simulink model "Estancia2024_2022a"  (R2022a)
settings: Solver=ode1  StartTime=0.0  StopTime=inf  FixedStep=0.0025  RelTol=1e-3  EnableMultiTasking=on
InitFcn:
  | Motor_Mapping_7_Inch
model workspace (MAT data in the model file):
  target_system = 1
values from neighbouring files (symbols this model uses):
  F1 = F1 + 2*(PSI_I'*C'*Q_z*C*PHI_I)    [Setup_MPC_SMC_Drone.m]
  F1_xy = F1_xy + 2*(PSI_xy_I'*C_xy'*Q_xy*C_xy*PHI_xy_I)    [Setup_MPC_SMC_Drone.m]
  F2 = F2 - 2*(PSI_I'*C'*Q_z*pi_n)    [Setup_MPC_SMC_Drone.m]
  F2_xy = F2_xy - 2*(PSI_xy_I'*C_xy'*Q_xy*pi_n)    [Setup_MPC_SMC_Drone.m]
  F3 = F3 - 2*(pi_nu'*Qt_z)    [Setup_MPC_SMC_Drone.m]
  F3_xy = F3_xy - 2*(pi_nu'*R_xy)    [Setup_MPC_SMC_Drone.m]
  F4 = F4 + 2*(PSI_I'*C'*Qt_z*C*SumG)    [Setup_MPC_SMC_Drone.m]
  G = [0;-g]    [Setup_MPC_SMC_Drone.m]
  H = H + 2*(PSI_I'*C'*Q_z*C*PSI_I + pi_nu'*Qt_z*pi_nu)    [Setup_MPC_SMC_Drone.m]
  H_xy = H_xy + 2*(PSI_xy_I'*C_xy'*Q_xy*C_xy*PSI_xy_I + pi_nu'*R_xy*pi_nu)    [Setup_MPC_SMC_Drone.m]
  J = diag([Jxx Jyy Jzz])    [Setup_MPC_SMC_Drone.m]
  m = 1.121    [Setup_MPC_SMC_Drone.m]
  N = 10    [Setup_MPC_SMC_Drone.m]
  N_xy = 10    [Setup_MPC_SMC_Drone.m]
  ny = size(C,1)    [Setup_MPC_SMC_Drone.m]
  ny_xy = size(C_xy,1)    [Setup_MPC_SMC_Drone.m]
  u_des = 0    [Setup_MPC_SMC_Drone.m]
  u_des_xy = [0;0]    [Setup_MPC_SMC_Drone.m]
undefined symbols (not defined in the file or in its folder): _Commander, _QDrone2, _Stabilizer, A_l, B_l, C_l, datetime, F1_l, F1_z, F2_l, F2_z, F3_l, F3_z, F4_z, H_l, H_z, HIL, KT, lf, log_, max_ul, min_ul, Motor_Matrix, n, N_l, N_z, nr_l, nr_z, nu, nu_l, nu_xy, nu_z, phi_l, psi_l, qc_get_step_size, Qu_l, Qy_l, s, saved_data, u_dz, ud_l
libraries: quarc_library x95, simulink x27, simulink_extras x10, matrix_library x1, aerolibutil x1
(part 4 of 5)

== system Estancia2024_2022a/COMMANDER (ANGLE MODE)/Subsystem/Z MPC ==
  pose : Inport
  pose_rate : Inport  Port=2
  ref : Inport  Port=3
  Add : Sum  Inputs=+++-
  Add1 : Sum
  Constant : Constant  Value=F1
  Constant1 : Constant  Value=F2
  Constant2 : Constant  Value=F3
  Constant3 : Constant  Value=F4
  Constant4 : Constant  Value=H
  Constant5 : Constant  Value=u_des
  Constant6 : Constant  Commented=on  Value=G
  Constant7 : Constant  Value=ones(1,N)
  Constant8 : Constant  Commented=on  Value=ones(2,N*2)
  Constant9 : Constant  Value=0.38
  MATLAB Function : MATLAB Function  TreatAsAtomicUnit=on
  MATLAB Function1 : MATLAB Function  Commented=on  TreatAsAtomicUnit=on
  MatrixMultiply{,1..3} (4 alike) : Product  Multiplication=Matrix(*)
  MatrixMultiply5 : Product  Commented=on  Multiplication=Matrix(*)
  Mux : Mux  Inputs=2
  Product : Product
  Reshape : Reshape  OutputDimensionality=Customize  OutputDimensions=[N*ny,1]
  Reshape1 : Reshape  Commented=on  OutputDimensionality=Customize  OutputDimensions=[2*N,1]
  Saturation : Saturate  UpperLimit=50  LowerLimit=0
  Scope : Scope
  Selector : Selector  InputPortWidth=N*nu  IndexOptions=Index vector (dialog)  Indices=1  OutputSizes=1
  Selector1 : Selector  InputPortWidth=4  IndexOptions=Index vector (dialog)  Indices=3  OutputSizes=1
  Selector2 : Selector  InputPortWidth=4  IndexOptions=Index vector (dialog)  Indices=3  OutputSizes=1
  Selector3 : Selector  InputPortWidth=4  IndexOptions=Index vector (dialog)  Indices=3  OutputSizes=1
  Thrust : Outport
  wires:
  Add/1 -> MATLAB Function/2(F)
  Constant4/1 -> MATLAB Function/1(H)
  MATLAB Function/1(u_opt) -> Selector/1
  Constant/1 -> MatrixMultiply/1
  MatrixMultiply/1 -> Add/1
  MatrixMultiply1/1 -> Add/2
  MatrixMultiply2/1 -> Add/3
  MatrixMultiply3/1 -> Add/4
  Mux/1 -> MatrixMultiply/2
  Selector2/1 -> Mux/2
  Selector1/1 -> Mux/1
  pose/1 -> Selector1/1
  Constant1/1 -> MatrixMultiply1/1
  Constant5/1 -> MatrixMultiply2/2
  Constant2/1 -> MatrixMultiply2/1
  Constant7/1 -> Product/2
  Selector3/1 -> Product/1
  Product/1 -> Reshape/1
  Reshape/1 -> MatrixMultiply1/2
  Constant8/1 -> MatrixMultiply5/2
  Constant6/1 -> MATLAB Function1/1(u)
  MatrixMultiply5/1 -> Reshape1/1
  Reshape1/1 -> MatrixMultiply3/2
  Constant3/1 -> MatrixMultiply3/1
  MATLAB Function1/1(y) -> MatrixMultiply5/1
  Add1/1 -> Selector3/1
  ref/1 -> Add1/1
  Constant9/1 -> Add1/2
  Selector/1 -> Saturation/1
  Saturation/1 -> Scope/1, Thrust/1
  pose_rate/1 -> Selector2/1

== system Estancia2024_2022a/COMMANDER (ANGLE MODE)/THROTTLE SWITCHBOX /Use desired height when enabled ==
  h_d (m) [1] : Inport
  Enable : EnablePort
  Out1 : Outport  OutputWhenDisabled=reset  InitialOutput=0  VectorParamsAs1DForOutWhenUnconnected=off
  wires:
  h_d (m) [1]/1 -> Out1/1

== system Estancia2024_2022a/HORIZON FRAME CONVERSION AND ESTIMATION/Pose Switchbox/Use des height when enabled ==
  h_d (m) [1] : Inport
  Enable : EnablePort
  Out1 : Outport  OutputWhenDisabled=reset  InitialOutput=0  VectorParamsAs1DForOutWhenUnconnected=off
  wires:
  h_d (m) [1]/1 -> Out1/1

== system Estancia2024_2022a/HORIZON FRAME CONVERSION AND ESTIMATION/Pose Switchbox/Use des yaw when enabled ==
  h_d (m) [1] : Inport
  Enable : EnablePort
  Out1 : Outport  OutputWhenDisabled=reset  InitialOutput=0  VectorParamsAs1DForOutWhenUnconnected=off
  wires:
  h_d (m) [1]/1 -> Out1/1

== system Estancia2024_2022a/HORIZON FRAME CONVERSION AND ESTIMATION/Pose Switchbox/Use desired X when enabled ==
  h_d (m) [1] : Inport
  Enable : EnablePort
  Out1 : Outport  OutputWhenDisabled=reset  InitialOutput=0  VectorParamsAs1DForOutWhenUnconnected=off
  wires:
  h_d (m) [1]/1 -> Out1/1

== system Estancia2024_2022a/HORIZON FRAME CONVERSION AND ESTIMATION/Pose Switchbox/Use desired Y when enabled ==
  h_d (m) [1] : Inport
  Enable : EnablePort
  Out1 : Outport  OutputWhenDisabled=reset  InitialOutput=0  VectorParamsAs1DForOutWhenUnconnected=off
  wires:
  h_d (m) [1]/1 -> Out1/1

== system Estancia2024_2022a/QDrone2 DAQ/Attitude Estimate from IMU Data/For Each Subsystem - Attitutde Estimates ==
  note: Attitude Estimates from IMU Data
  note: Accelerometer (m/s/s) [3]
  note: Roll And Pitch From Accelerometer Filter + Attitude Approximation
  note: Roll & Pitch angle estimation via sensor fusion
  note: Angular Acceleration Estimation via Filter + Derivative
  "IMU (rad/s, m/s^2) [6n]" : Inport  Partition=on  PartitionDimension=1  PartitionWidth=6  PartitionOffset=0
  Constant : Constant  Value=120
  Constant10 : Constant  Value=0.7
  Constant3 : Constant
  Constant9 : Constant  Value=100
  Demux : Demux  Outputs=[3,3]
  For Each : ForEach  DisableCoverage=on
  Integrator2 : Integrator
  Integrator3 : Integrator
  Integrator4 : Integrator
  Ki1 : Gain  Gain=[0.1 0.1]
  Kp1 : Gain  Gain=[0.25 0.25]
  Mux : Mux  Inputs=3
  Mux4 : Mux  Inputs=2
  Mux5 : Mux  Inputs=2
  Second-Order Low-Pass Filter (Roll and Pitch Rate) : quarc_library/Continuous/Second-Order Low-Pass Filter  params_source=External (input ports)  input_width=200  input_zeta=1  input_init=0
  Second-Order Low-Pass Filter (Yaw Rate) : quarc_library/Continuous/Second-Order Low-Pass Filter  params_source=External (input ports)  input_width=200  input_zeta=1  input_init=0
  Selector2 : Selector  InputPortWidth=3  IndexOptions=Index vector (dialog)  Indices=[1,2]  OutputSizes=1
  Selector3 : Selector  InputPortWidth=3  IndexOptions=Index vector (dialog)  Indices=[3]  OutputSizes=1
  Sum1 : Sum  Inputs=+--
  Sum4 : Sum  Inputs=|-+
  Terminator1 : Terminator
  roll and pitch approximation from accelerometer : MATLAB Function  TreatAsAtomicUnit=on
  BF Att (rad) [3n] : Outport  ConcatenationDimension=1
  BF Att Rate (rad/s) [3n] : Outport  Port=2  ConcatenationDimension=1
  BF Att Accel (rad/s^2) [3n] : Outport  Port=3  ConcatenationDimension=1
  "BF Estimated Att (rad, rad/s, rad/s^2) [9n] " : Outport  Port=4  ConcatenationDimension=1
  wires:
  roll and pitch approximation from accelerometer/2(pitch_acc) -> Mux4/2
  Constant9/1 -> Second-Order Low-Pass Filter (Roll and Pitch Rate)/2
  Second-Order Low-Pass Filter (Roll and Pitch Rate)/1 -> roll and pitch approximation from accelerometer/1(acc_body)
  "IMU (rad/s, m/s^2) [6n]"/1 -> Demux/1  "IMU 0 Data (rad/s,m/s^2)"
  Constant10/1 -> Second-Order Low-Pass Filter (Roll and Pitch Rate)/3
  Demux/2 -> Second-Order Low-Pass Filter (Roll and Pitch Rate)/4, Second-Order Low-Pass Filter (Roll and Pitch Rate)/1
  Second-Order Low-Pass Filter (Roll and Pitch Rate)/2 -> Terminator1/1
  Selector3/1 -> Integrator2/1
  Integrator2/1 -> Mux5/2
  Integrator4/1 -> Sum1/3
  Kp1/1 -> Sum1/2
  Selector2/1 -> Sum1/1
  Integrator3/1 -> Sum4/2, Mux5/1
  Mux5/1 -> BF Att (rad) [3n]/1, Mux/1
  Sum4/1 -> Ki1/1, Kp1/1
  Sum1/1 -> Integrator3/1
  Ki1/1 -> Integrator4/1
  roll and pitch approximation from accelerometer/1(roll_acc) -> Mux4/1
  Mux4/1 -> Sum4/1
  Constant3/1 -> Second-Order Low-Pass Filter (Yaw Rate)/3
  Demux/1 -> Second-Order Low-Pass Filter (Yaw Rate)/4, Second-Order Low-Pass Filter (Yaw Rate)/1, Selector3/1, Selector2/1  "BF Gyroscope Data (rad/s)"
  Constant/1 -> Second-Order Low-Pass Filter (Yaw Rate)/2
  Second-Order Low-Pass Filter (Yaw Rate)/1 -> Mux/2, BF Att Rate (rad/s) [3n]/1
  Second-Order Low-Pass Filter (Yaw Rate)/2 -> BF Att Accel (rad/s^2) [3n]/1, Mux/3  "BF Angular Accel. Estimates (rad/s/s) [3]"
  Mux/1 -> "BF Estimated Att (rad, rad/s, rad/s^2) [9n] "/1

== system Estancia2024_2022a/QDrone2 DAQ/Check Battery level/Triggered Subsystem ==
  Trigger : TriggerPort  VariantControl=(inherit)
  Constant : Constant
  Out1 : Outport  InitialOutput=[0]
  wires:
  Constant/1 -> Out1/1

== system Estancia2024_2022a/QDrone2 DAQ/Sensor Failure Monitoring - IMU0/Sensor Failure (Accelerometer) ==
  note: Check for flat-line ZERO Accelerometer data (no data)
  Sensor Input : Inport
  Clock : Clock
  Compare To Constant : simulink/Logic and Bit Operations/Compare To Constant  relop=>=  const=1  OutDataTypeStr=boolean
  Demux1 : Demux  Outputs=3
  Logical Operator : Logic  Operator=OR  Inputs=3  AllPortsSameDT=off  OutDataTypeStr=boolean
  Logical Operator1 : Logic  AllPortsSameDT=off  OutDataTypeStr=boolean
  Terminator1 : Terminator
  Terminator3 : Terminator
  Terminator4 : Terminator
  Threshold : quarc_library/Discontinuities/Threshold  operator===  param_src=Specify via dialog  threshold=0  duration=1
      settings: SourceProductName=QUARC Targets
  Threshold1 : quarc_library/Discontinuities/Threshold  operator===  param_src=Specify via dialog  threshold=0  duration=1
      settings: SourceProductName=QUARC Targets
  Threshold2 : quarc_library/Discontinuities/Threshold  operator===  param_src=Specify via dialog  threshold=0  duration=1
      settings: SourceProductName=QUARC Targets
  Sensor Fault : Outport  VectorParamsAs1DForOutWhenUnconnected=off
  wires:
  Clock/1 -> Compare To Constant/1
  Threshold/1 -> Logical Operator/1
  Threshold1/1 -> Logical Operator/2
  Compare To Constant/1 -> Logical Operator1/1
  Logical Operator1/1 -> Sensor Fault/1
  Sensor Input/1 -> Demux1/1
  Threshold2/2 -> Terminator4/1
  Threshold2/1 -> Logical Operator/3
  Demux1/1 -> Threshold/1
  Demux1/3 -> Threshold2/1
  Demux1/2 -> Threshold1/1
  Logical Operator/1 -> Logical Operator1/2
  Threshold1/2 -> Terminator3/1
  Threshold/2 -> Terminator1/1

== system Estancia2024_2022a/QDrone2 DAQ/Sensor Failure Monitoring - IMU0/Sensor Failure (Gyroscope) ==
  note: Check for flat-line ZERO Gyro data (no data)
  Sensor Input : Inport
  Clock : Clock
  Compare To Constant : simulink/Logic and Bit Operations/Compare To Constant  relop=>=  const=1  OutDataTypeStr=boolean
  Demux1 : Demux  Outputs=3
  Logical Operator : Logic  Operator=OR  Inputs=3  AllPortsSameDT=off  OutDataTypeStr=boolean
  Logical Operator1 : Logic  AllPortsSameDT=off  OutDataTypeStr=boolean
  Terminator1 : Terminator
  Terminator3 : Terminator
  Terminator4 : Terminator
  Threshold : quarc_library/Discontinuities/Threshold  operator===  param_src=Specify via dialog  threshold=0  duration=1
      settings: SourceProductName=QUARC Targets
  Threshold1 : quarc_library/Discontinuities/Threshold  operator===  param_src=Specify via dialog  threshold=0  duration=1
      settings: SourceProductName=QUARC Targets
  Threshold2 : quarc_library/Discontinuities/Threshold  operator===  param_src=Specify via dialog  threshold=0  duration=1
      settings: SourceProductName=QUARC Targets
  Sensor Fault : Outport  VectorParamsAs1DForOutWhenUnconnected=off
  wires:
  Threshold/2 -> Terminator1/1
  Threshold1/2 -> Terminator3/1
  Logical Operator/1 -> Logical Operator1/2
  Demux1/2 -> Threshold1/1
  Demux1/3 -> Threshold2/1
  Demux1/1 -> Threshold/1
  Threshold2/1 -> Logical Operator/3
  Threshold2/2 -> Terminator4/1
  Sensor Input/1 -> Demux1/1
  Logical Operator1/1 -> Sensor Fault/1
  Compare To Constant/1 -> Logical Operator1/1
  Threshold1/1 -> Logical Operator/2
  Threshold/1 -> Logical Operator/1
  Clock/1 -> Compare To Constant/1

== system Estancia2024_2022a/QDrone2 DAQ/Sensor Failure Monitoring - IMU1/Sensor Failure (Accelerometer) ==
  note: Check for flat-line ZERO Accelerometer data (no data)
  Sensor Input : Inport
  Clock : Clock
  Compare To Constant : simulink/Logic and Bit Operations/Compare To Constant  relop=>=  const=1  OutDataTypeStr=boolean
  Demux1 : Demux  Outputs=3
  Logical Operator : Logic  Operator=OR  Inputs=3  AllPortsSameDT=off  OutDataTypeStr=boolean
  Logical Operator1 : Logic  AllPortsSameDT=off  OutDataTypeStr=boolean
  Terminator1 : Terminator
  Terminator3 : Terminator
  Terminator4 : Terminator
  Threshold : quarc_library/Discontinuities/Threshold  operator===  param_src=Specify via dialog  threshold=0  duration=1
      settings: SourceProductName=QUARC Targets
  Threshold1 : quarc_library/Discontinuities/Threshold  operator===  param_src=Specify via dialog  threshold=0  duration=1
      settings: SourceProductName=QUARC Targets
  Threshold2 : quarc_library/Discontinuities/Threshold  operator===  param_src=Specify via dialog  threshold=0  duration=1
      settings: SourceProductName=QUARC Targets
  Sensor Fault : Outport  VectorParamsAs1DForOutWhenUnconnected=off
  wires:
  Threshold/2 -> Terminator1/1
  Threshold1/2 -> Terminator3/1
  Logical Operator/1 -> Logical Operator1/2
  Demux1/2 -> Threshold1/1
  Demux1/3 -> Threshold2/1
  Demux1/1 -> Threshold/1
  Threshold2/1 -> Logical Operator/3
  Threshold2/2 -> Terminator4/1
  Sensor Input/1 -> Demux1/1
  Logical Operator1/1 -> Sensor Fault/1
  Compare To Constant/1 -> Logical Operator1/1
  Threshold1/1 -> Logical Operator/2
  Threshold/1 -> Logical Operator/1
  Clock/1 -> Compare To Constant/1

== system Estancia2024_2022a/QDrone2 DAQ/Sensor Failure Monitoring - IMU1/Sensor Failure (Gyroscope) ==
  note: Check for flat-line ZERO Gyro data (no data)
  Sensor Input : Inport
  Clock : Clock
  Compare To Constant : simulink/Logic and Bit Operations/Compare To Constant  relop=>=  const=1  OutDataTypeStr=boolean
  Demux1 : Demux  Outputs=3
  Logical Operator : Logic  Operator=OR  Inputs=3  AllPortsSameDT=off  OutDataTypeStr=boolean
  Logical Operator1 : Logic  AllPortsSameDT=off  OutDataTypeStr=boolean
  Terminator1 : Terminator
  Terminator3 : Terminator
  Terminator4 : Terminator
  Threshold : quarc_library/Discontinuities/Threshold  operator===  param_src=Specify via dialog  threshold=0  duration=1
      settings: SourceProductName=QUARC Targets
  Threshold1 : quarc_library/Discontinuities/Threshold  operator===  param_src=Specify via dialog  threshold=0  duration=1
      settings: SourceProductName=QUARC Targets
  Threshold2 : quarc_library/Discontinuities/Threshold  operator===  param_src=Specify via dialog  threshold=0  duration=1
      settings: SourceProductName=QUARC Targets
  Sensor Fault : Outport  VectorParamsAs1DForOutWhenUnconnected=off
  wires:
  Clock/1 -> Compare To Constant/1
  Threshold/1 -> Logical Operator/1
  Threshold1/1 -> Logical Operator/2
  Compare To Constant/1 -> Logical Operator1/1
  Logical Operator1/1 -> Sensor Fault/1
  Sensor Input/1 -> Demux1/1
  Threshold2/2 -> Terminator4/1
  Threshold2/1 -> Logical Operator/3
  Demux1/1 -> Threshold/1
  Demux1/3 -> Threshold2/1
  Demux1/2 -> Threshold1/1
  Logical Operator/1 -> Logical Operator1/2
  Threshold1/2 -> Terminator3/1
  Threshold/2 -> Terminator1/1

== system Estancia2024_2022a/QDrone2 DAQ/Subsystem1/Maintain previous value4 ==
  Value in : Inport
  Memory : Memory
  Switch : Switch  Criteria=u2 ~= 0  SaturateOnIntegerOverflow=off  InputSameDT=off
  Non 0 values : Outport
  wires:
  Value in/1 -> Switch/1, Switch/2
  Switch/1 -> Memory/1, Non 0 values/1
  Memory/1 -> Switch/3

== system Estancia2024_2022a/STABILIZER - QDRONE 2/SMC ATTITUDE Controller/NFTSMC ==
  ref_angles : Inport
  pose : Inport  Port=2
  Constant : Constant  Value=J
  Derivative1 : Derivative
  Derivative4 : Derivative
  NFTSMC_ATTITUDE2 : Subsystem
  Scope : Scope
  Scope1 : Scope
  Selector11 : Selector  InputPortWidth=6  IndexOptions=Starting index (dialog)  Indices=[1]  OutputSizes=3
  Selector12 : Selector  InputPortWidth=6  IndexOptions=Starting index (dialog)  Indices=[4]  OutputSizes=3
  Selector13 : Selector  InputPortWidth=6  IndexOptions=Starting index (dialog)  Indices=[4]  OutputSizes=3
  Sum1 : Sum  Inputs=+-|
  Sum4 : Sum  Inputs=+-|
  torques : Outport
  wires:
  Sum4/1 -> Scope1/1, NFTSMC_ATTITUDE2/2(e_dot)  "e_dot"
  Sum1/1 -> Scope/1, NFTSMC_ATTITUDE2/1(e)  "e"
  Selector11/1 -> Sum1/1
  Selector13/1 -> NFTSMC_ATTITUDE2/5(w)
  Selector12/1 -> Sum4/1
  pose/1 -> Selector11/1, Selector12/1, Selector13/1
  Constant/1 -> NFTSMC_ATTITUDE2/4(J)
  NFTSMC_ATTITUDE2/1(torques) -> torques/1
  Derivative4/1 -> NFTSMC_ATTITUDE2/3(w_dot)
  Derivative1/1 -> Derivative4/1, Sum4/2
  ref_angles/1 -> Derivative1/1, Sum1/2

== system Estancia2024_2022a/COMMANDER (ANGLE MODE)/MPC/Lineal MPC1/For Iterator Subsystem ==
  x_k : Inport
  y_d : Inport  Port=2
  u_d : Inport  Port=3
  Add8 : Sum  Inputs=+++
  Constant11 : Constant  Value=phi_l
  Constant12 : Constant  Value=psi_l
  Constant13 : Constant  Value=C_l
  Constant14 : Constant  Value=Qy_l
  Constant16 : Constant  Value=N_l
  Constant2 : Constant  Value=B_l
  Constant3 : Constant  Value=A_l
  Constant5 : Constant  Value=Qu_l
  MATLAB Function : MATLAB Function  TreatAsAtomicUnit=on
  Matrix Multiply5 : Product  Multiplication=Matrix(*)
  Matrix Multiply6 : Product  Multiplication=Matrix(*)
  Matrix Multiply7 : Product  Multiplication=Matrix(*)
  Nr : Constant  Value=eye(nr_l*N_l,nr_l*N_l)
  Nu : Constant  Value=eye(nu_l*N_l,nu_l*N_l)
  H : Outport
  F : Outport  Port=2
  wires:
  x_k/1 -> Matrix Multiply5/2
  y_d/1 -> Matrix Multiply6/2
  u_d/1 -> Matrix Multiply7/2
  Matrix Multiply6/1 -> Add8/2
  Matrix Multiply5/1 -> Add8/1
  Matrix Multiply7/1 -> Add8/3
  Add8/1 -> F/1
  Nr/1 -> MATLAB Function/9(Pi_nr)
  Nu/1 -> MATLAB Function/8(Pi_nu)
  Constant16/1 -> MATLAB Function/10(N)
  Constant11/1 -> MATLAB Function/1(phi)
  Constant14/1 -> MATLAB Function/6(Qy)
  Constant12/1 -> MATLAB Function/2(psi)
  Constant13/1 -> MATLAB Function/5(C)
  Constant2/1 -> MATLAB Function/4(B)
  Constant3/1 -> MATLAB Function/3(A)
  MATLAB Function/4(F3) -> Matrix Multiply7/1
  MATLAB Function/3(F2) -> Matrix Multiply6/1
  MATLAB Function/2(F1) -> Matrix Multiply5/1
  MATLAB Function/1(H) -> H/1
  Constant5/1 -> MATLAB Function/7(Qu)

== system Estancia2024_2022a/COMMANDER (ANGLE MODE)/STATE MACHINE SIGNALS/Generate Extra Messages for Console/Boolean Edge-Based Triggered Print ==
  Signal Enable : Inport  Partition=on  PartitionDimension=1  PartitionWidth=1  PartitionOffset=0
  Message : Inport  Port=2  Partition=on  PartitionDimension=2  PartitionWidth=1  PartitionOffset=0
  time (s) : Inport  Port=3
  For Each : ForEach  DisableCoverage=on
  Triggered Subsystem1 : Subsystem  TreatAsAtomicUnit=on
  Out1 : Outport  ConcatenationDimension=1
  wires:
  time (s)/1 -> Triggered Subsystem1/1(Time (s))
  Message/1 -> Triggered Subsystem1/2(Message)
  Signal Enable/1 -> Out1/1, Triggered Subsystem1/Trigger

== system Estancia2024_2022a/COMMANDER (ANGLE MODE)/STATE MACHINE SIGNALS/Generate State Messages for Console/Triggered Subsystem ==
  Value : Inport
  Time (s) : Inport  Port=2
  Message : Inport  Port=3
  Trigger : TriggerPort  VariantControl=(inherit)
  Data Type Conversion : DataTypeConversion  OutDataTypeStr=uint8  SaturateOnIntegerOverflow=off  RndMeth=Floor
  Print : quarc_library/User Interface/Standard I//O/Print  format_string="[ %lf ] (s): State %u  => %s \\n"  max_code_units=512  optimization=Minimizing latency  sample_time=-1  active=off
      settings: SourceProductName=QUARC Targets
  Terminator : Terminator
  Terminator1 : Terminator
  wires:
  Time (s)/1 -> Print/1
  Message/1 -> Print/3
  Print/2 -> Terminator/1
  Print/1 -> Terminator1/1
  Value/1 -> Data Type Conversion/1
  Data Type Conversion/1 -> Print/2

== system Estancia2024_2022a/COMMANDER (ANGLE MODE)/STATE MACHINE SIGNALS/Generate Warning Messages for Console/Boolean Value-Based Triggered Print ==
  Signal Enable : Inport  Partition=on  PartitionDimension=1  PartitionWidth=1  PartitionOffset=0
  Message : Inport  Port=2  Partition=on  PartitionDimension=2  PartitionWidth=1  PartitionOffset=0
  time (s) : Inport  Port=3
  For Each : ForEach  DisableCoverage=on
  Triggered Subsystem : Subsystem  TreatAsAtomicUnit=on
  Out1 : Outport  ConcatenationDimension=1
  wires:
  time (s)/1 -> Triggered Subsystem/1(Time (s))
  Message/1 -> Triggered Subsystem/2(Message)
  Signal Enable/1 -> Triggered Subsystem/Trigger, Out1/1

== system Estancia2024_2022a/STABILIZER - QDRONE 2/SMC ATTITUDE Controller/NFTSMC/NFTSMC_ATTITUDE2 ==
  e : Inport
  e_dot : Inport  Port=2
  w_dot : Inport  Port=3
  J : Inport  Port=4
  w : Inport  Port=5
  Add : Sum  Inputs=++--
  B/n + Ua : Subsystem
  Cross Product : matrix_library/Cross Product
  Invert 3x3 Matrix : aerolibutil/Invert  3x3 Matrix
  Matrix Multiply : Product  Multiplication=Matrix(*)
  Matrix Multiply1 : Product  Multiplication=Matrix(*)
  Matrix Multiply2 : Product  Multiplication=Matrix(*)
  torques : Outport
  wires:
  J/1 -> [J], Matrix Multiply1/1, Invert 3x3 Matrix/1
  Invert 3x3 Matrix/1 -> Matrix Multiply/1
  Cross Product/1 -> Matrix Multiply/2
  Matrix Multiply1/1 -> Cross Product/2
  w/1 -> [w], Matrix Multiply1/2
  [w] -> Cross Product/1
  w_dot/1 -> Add/1
  Matrix Multiply/1 -> Add/2
  Add/1 -> Matrix Multiply2/2
  Matrix Multiply2/1 -> torques/1
  [J] -> Matrix Multiply2/1
  B/n + Ua/1(Bn) -> Add/3
  B/n + Ua/2(Ua) -> Add/4
  e_dot/1 -> B/n + Ua/1(e_dot)
  e/1 -> B/n + Ua/2(e)

== system Estancia2024_2022a/COMMANDER (ANGLE MODE)/STATE MACHINE SIGNALS/Generate Extra Messages for Console/Boolean Edge-Based Triggered Print/Triggered Subsystem1 ==
  Time (s) : Inport
  Message : Inport  Port=2
  Trigger : TriggerPort  TriggerType=falling  VariantControl=(inherit)
  Print : quarc_library/User Interface/Standard I//O/Print  format_string=[ %lf ] (s): %s !\n  max_code_units=512  optimization=Minimizing latency  sample_time=-1  active=off
      settings: SourceProductName=QUARC Targets
  Terminator : Terminator
  Terminator1 : Terminator
  wires:
  Time (s)/1 -> Print/1
  Message/1 -> Print/2
  Print/2 -> Terminator/1
  Print/1 -> Terminator1/1

== system Estancia2024_2022a/COMMANDER (ANGLE MODE)/STATE MACHINE SIGNALS/Generate Warning Messages for Console/Boolean Value-Based Triggered Print/Triggered Subsystem ==
  Time (s) : Inport
  Message : Inport  Port=2
  Trigger : TriggerPort  VariantControl=(inherit)
  Print : quarc_library/User Interface/Standard I//O/Print  format_string=[ %lf ] (s): %s\n  max_code_units=512  optimization=Minimizing latency  sample_time=-1  active=off
      settings: SourceProductName=QUARC Targets
  Terminator : Terminator
  Terminator1 : Terminator
  wires:
  Print/1 -> Terminator1/1
  Print/2 -> Terminator/1
  Message/1 -> Print/2
  Time (s)/1 -> Print/1

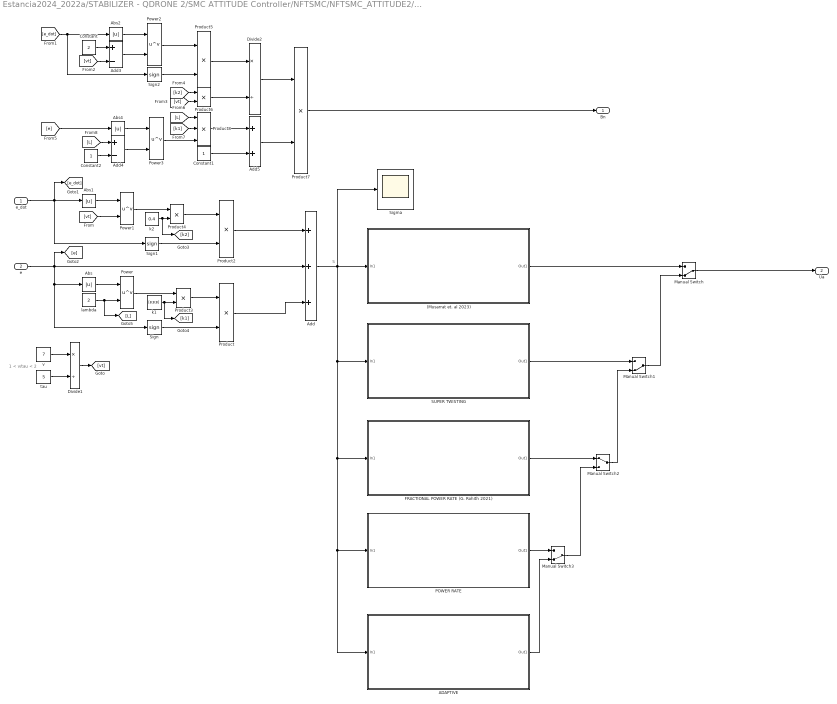
== system Estancia2024_2022a/STABILIZER - QDRONE 2/SMC ATTITUDE Controller/NFTSMC/NFTSMC_ATTITUDE2/B//n + Ua ==
  note: S
  note: 1 < v/tau < 2
  e_dot : Inport
  e : Inport  Port=2
  " (Musarrat et. al 2023)" : Subsystem
  ADAPTIVE : Subsystem
  Abs{,1..2,4} (4 alike) : Abs  SaturateOnIntegerOverflow=off
  Add : Sum  Inputs=+++
  Add3 : Sum  Inputs=+-
  Add4 : Sum  Inputs=+-
  Add5 : Sum
  Constant : Constant  Value=2
  Constant1 : Constant
  Constant2 : Constant
  Divide1 : Product  Inputs=*/
  Divide2 : Product  Inputs=*/
  FRACTIONAL POWER RATE (G. Rohith 2021) : Subsystem
  Manual Switch : ManualSwitch  CurrentSetting=0
  Manual Switch1 : ManualSwitch  CurrentSetting=0
  Manual Switch2 : ManualSwitch
  Manual Switch3 : ManualSwitch  CurrentSetting=0
  POWER RATE : Subsystem
  Power{,1..3} (4 alike) : Math  Operator=pow
  Product{,2..7} (7 alike) : Product
  Product8 : Product  Inputs=3
  SUPER TWISTING : Subsystem
  Sigma : Scope
  Sign : Signum
  Sign1 : Signum
  Sign2 : Signum
  k1 : Constant  Value=[8;8;8]
  k2 : Constant  Value=0.4  VectorParams1D=off
  lambda : Constant  Value=2
  tau : Constant  Value=5
  v : Constant  Value=7
  Bn : Outport
  Ua : Outport  Port=2
  wires:
  Constant1/1 -> Add5/2
  [k2] -> Product6/1
  Power3/1 -> Product8/3
  Product5/1 -> Divide2/1
  Product6/1 -> Divide2/2
  k1/1 -> Product3/2, [k1]
  tau/1 -> Divide1/2
  lambda/1 -> [L], Power/2
  [vt] -> Power1/2
  [vt] -> Product6/2
  [e_dot] -> Sign2/1, Abs2/1
  Power1/1 -> Product4/1
  Sign1/1 -> Product2/2
  Add4/1 -> Power3/2
  [k1] -> Product8/2
  Product/1 -> Add/3
  e/1 -> [e], Abs/1, Sign/1, Add/2
  Constant2/1 -> Add4/2
  v/1 -> Divide1/1
  Sign/1 -> Product/2
  k2/1 -> [k2], Product4/2
  Sign2/1 -> Product5/2
  Add3/1 -> Power2/2
  Power2/1 -> Product5/1
  Abs2/1 -> Power2/1
  Abs/1 -> Power/1
  Constant/1 -> Add3/1
  [vt] -> Add3/2
  [L] -> Add4/1
  Abs1/1 -> Power1/1
  [L] -> Product8/1
  e_dot/1 -> [e_dot], Abs1/1, Sign1/1
  Add5/1 -> Product7/2
  [e] -> Abs4/1
  Divide2/1 -> Product7/1
  Product3/1 -> Product/1
  Power/1 -> Product3/1
  Product8/1 -> Add5/1
  Product2/1 -> Add/1
  Abs4/1 -> Power3/1
  Product4/1 -> Product2/1
  Divide1/1 -> [vt]
  Product7/1 -> Bn/1
  Add/1 -> Sigma/1, SUPER TWISTING/1(In1), ADAPTIVE/1(In1), POWER RATE/1(In1), FRACTIONAL POWER RATE (G. Rohith 2021)/1(In1), " (Musarrat et. al 2023)"/1(In1)
  " (Musarrat et. al 2023)"/1(Out1) -> Manual Switch/1
  Manual Switch/1 -> Ua/1
  SUPER TWISTING/1(Out1) -> Manual Switch1/1
  Manual Switch1/1 -> Manual Switch/2
  FRACTIONAL POWER RATE (G. Rohith 2021)/1(Out1) -> Manual Switch2/1
  Manual Switch2/1 -> Manual Switch1/2
  POWER RATE/1(Out1) -> Manual Switch3/1
  ADAPTIVE/1(Out1) -> Manual Switch3/2
  Manual Switch3/1 -> Manual Switch2/2

== system Estancia2024_2022a/STABILIZER - QDRONE 2/SMC ATTITUDE Controller/NFTSMC/NFTSMC_ATTITUDE2/B//n + Ua/ (Musarrat et. al 2023) ==
  In1 : Inport
  Abs3 : Abs  SaturateOnIntegerOverflow=off
  Add2 : Sum
  Power4 : Math  Operator=pow
  Power6 : Math  Operator=pow
  Product1 : Product  Inputs=3
  Product9 : Product  Inputs=3
  Sign3 : Signum
  Sign5 : Signum
  c1 : Constant  Value=0.1
  c2 : Constant  Value=1.1
  y1 : Constant  Value=7
  y2 : Constant  Value=5
  Out1 : Outport
  wires:
  Add2/1 -> Out1/1
  Product1/1 -> Add2/2
  y2/1 -> Product1/2
  c1/1 -> Power4/2
  Power4/1 -> Product9/3
  Abs3/1 -> Power4/1, Power6/1
  Sign5/1 -> Product1/3
  Sign3/1 -> Product9/1
  In1/1 -> Sign5/1, Sign3/1, Abs3/1
  Power6/1 -> Product1/1
  Product9/1 -> Add2/1
  c2/1 -> Power6/2
  y1/1 -> Product9/2

== system Estancia2024_2022a/STABILIZER - QDRONE 2/SMC ATTITUDE Controller/NFTSMC/NFTSMC_ATTITUDE2/B//n + Ua/ADAPTIVE ==
  In1 : Inport
  Abs : Abs  SaturateOnIntegerOverflow=off
  Add : Sum
  Gain : Gain  Gain=0.01
  Integrator : Integrator  InitialCondition=20
  Lambda : Constant  Value=2
  Product : Product
  Product1 : Product
  Scope : Scope
  Tanh : Trigonometry  Operator=tanh
  Out1 : Outport
  wires:
  In1/1 -> Tanh/1, Gain/1, Abs/1
  Abs/1 -> Product/2
  Lambda/1 -> Product/1
  Product/1 -> Integrator/1
  Gain/1 -> Add/2
  Add/1 -> Scope/1, Out1/1
  Product1/1 -> Add/1
  Integrator/1 -> Product1/2
  Tanh/1 -> Product1/1

== system Estancia2024_2022a/STABILIZER - QDRONE 2/SMC ATTITUDE Controller/NFTSMC/NFTSMC_ATTITUDE2/B//n + Ua/FRACTIONAL POWER RATE (G. Rohith 2021) ==
  note: Ki = k/b
  In1 : Inport
  Abs3 : Abs  SaturateOnIntegerOverflow=off
  Add : Sum
  Add1 : Sum
  Divide : Product  Inputs=*/
  Gain : Gain  Gain=30
  Power1 : Math  Operator=pow
  Power4 : Math  Operator=pow
  Product1 : Product
  Product2 : Product
  Scope : Scope
  Sign : Signum
  b : Constant  Value=0.5
  c1 : Constant  Value=0.5
  k : Constant  Value=[5;5;5]
  sigma : Constant  Value=0.09
  Out1 : Outport
  wires:
  Power4/1 -> Product2/2
  c1/1 -> Power4/2
  Sign/1 -> Product2/1
  Abs3/1 -> Power1/2, Power4/1
  Product2/1 -> Product1/1
  sigma/1 -> Power1/1
  Power1/1 -> Add/1
  k/1 -> Divide/1
  Add/1 -> Divide/2
  Divide/1 -> Scope/1, Product1/2
  b/1 -> Add/2
  Product1/1 -> Add1/1
  Add1/1 -> Out1/1
  In1/1 -> Gain/1, Sign/1, Abs3/1
  Gain/1 -> Add1/2

== system Estancia2024_2022a/STABILIZER - QDRONE 2/SMC ATTITUDE Controller/NFTSMC/NFTSMC_ATTITUDE2/B//n + Ua/POWER RATE ==
  In1 : Inport
  Abs3 : Abs  SaturateOnIntegerOverflow=off
  Power4 : Math  Operator=pow
  Product9 : Product  Inputs=3
  Sign3 : Signum
  c1 : Constant  Value=0.5
  y1 : Constant  Value=5
  Out1 : Outport
  wires:
  Product9/1 -> Out1/1
  c1/1 -> Power4/2
  Power4/1 -> Product9/3
  Abs3/1 -> Power4/1
  Sign3/1 -> Product9/1
  In1/1 -> Sign3/1, Abs3/1
  y1/1 -> Product9/2

== system Estancia2024_2022a/STABILIZER - QDRONE 2/SMC ATTITUDE Controller/NFTSMC/NFTSMC_ATTITUDE2/B//n + Ua/SUPER TWISTING ==
  In1 : Inport
  Abs3 : Abs  SaturateOnIntegerOverflow=off
  Add : Sum
  Divide : Product  Inputs=*/
  Product2 : Product
  d : Constant  Value=0.5
  k1 : Constant  Value=20
  Out1 : Outport
  wires:
  k1/1 -> Product2/2
  Product2/1 -> Out1/1
  In1/1 -> Divide/1, Abs3/1
  Abs3/1 -> Add/2
  d/1 -> Add/1
  Add/1 -> Divide/2
  Divide/1 -> Product2/1

== matlab function Estancia2024_2022a/HORIZON FRAME CONVERSION AND ESTIMATION/Pose Switchbox/MATLAB Function2 ==
  data: sigmoid_type input; enable output; height_des input; slow_lim input; fast_lim input; height_cur input; height_vel input; height_ref output; max_height_vel output; max_height_accel output
function [enable, height_ref, max_height_vel, max_height_accel] = fcn(sigmoid_type, height_des, slow_lim, fast_lim, height_cur, height_vel)

% Note: Some of the cases below are identical. However, they are separated out 
% based on the states of the state machine for ease of modification in the future. 
% For example, states 4 and 5 are identical. However, if the user wants different 
% signmoid behaviour when taking off than when landing, these cases may not be the same. 

enable = 0;
height_ref = 0;
max_height_vel = 0;
max_height_accel = 0;

switch sigmoid_type
    case 1 % This is for the IDLE, ARM, E_ABORT, E_STOP and DISABLE states of the FSM
        enable = 0;
        height_ref = 0;
        max_height_vel = 0;
        max_height_accel = 0;

    case 2 % This is for the TAKEOFF THROTTLE state of the FSM
        enable = 0;
        height_ref = 0;
        max_height_vel = 0;
        max_height_accel = 0;

    case 3 % This is for the FLIGHT state of the FSM 
        enable = 1;
        height_ref = height_des;
        max_height_vel = fast_lim(1);
        max_height_accel = fast_lim(2);

    case 4 % This is for the TAKEOFF HEIGHT state of the FSM
        enable = 1;
        height_ref = height_des;
        if (height_vel < 0)||(abs(height_cur - height_des) <= 0.1)||(height_des <= height_cur)
            max_height_vel = fast_lim(1);
            max_height_accel = fast_lim(2);
        else    
            max_height_vel = slow_lim(1);
            max_height_accel = slow_lim(2);
        end
    case 5 % This is for the AUTOLAND state of the FSM
        enable = 1;
        height_ref = 0;
        if height_vel >= 0
            max_height_vel = fast_lim(1);
            max_height_accel = fast_lim(2);        
        else
            max_height_vel = slow_lim(1);
            max_height_accel = slow_lim(2);
        end
        
end

== matlab function Estancia2024_2022a/HORIZON FRAME CONVERSION AND ESTIMATION/Pose Switchbox/MATLAB Function4 ==
  data: sigmoid_type input; enable output; yaw_des input; slow_lim input; fast_lim input; yaw_cur input; yaw_ref output; max_yaw_vel output; max_yaw_accel output; yaw_vel input
function [enable, yaw_ref, max_yaw_vel, max_yaw_accel] = fcn(sigmoid_type, yaw_des, slow_lim, fast_lim, yaw_cur, yaw_vel)

% Note: Some of the cases below are identical. However, they are separated out 
% based on the states of the state machine for ease of modification in the future. 
% For example, states 4 and 5 are identical. However, if the user wants different 
% signmoid behaviour when taking off than when landing, these cases may not be the same. 

enable = 0;
yaw_ref = 0;
max_yaw_vel = 0;
max_yaw_accel = 0;

switch sigmoid_type
    case 1 % This is for the IDLE, ARM, E_ABORT, E_STOP and DISABLE states of the FSM
        enable = 0;
        yaw_ref = 0;
        max_yaw_vel = 0;
        max_yaw_accel = 0;
    case 2 % This is for the TAKEOFF THROTTLE state of the FSM
        enable = 1;
        yaw_ref = yaw_des;
        max_yaw_vel = slow_lim(1);
        max_yaw_accel = slow_lim(2);  
    case 3 % This is for the FLIGHT state of the FSM 
        enable = 1;
        yaw_ref = yaw_des;
        max_yaw_vel = fast_lim(1);
        max_yaw_accel = fast_lim(2);
    case 4 % This is for the TAKEOFF HEIGHT state of the FSM
        enable = 1;
        yaw_ref = yaw_des;
        if (yaw_vel < 0)||(yaw_des < yaw_cur)||(abs(yaw_cur-yaw_des)<=0.2)
            max_yaw_vel = fast_lim(1);
            max_yaw_accel = fast_lim(2);
        else    
            max_yaw_vel = slow_lim(1);
            max_yaw_accel = slow_lim(2);
        end
    case 5 % This is for the AUTOLAND state of the FSM
        enable = 1;
        yaw_ref = yaw_des;
        if (yaw_vel >= 0)
            max_yaw_vel = fast_lim(1);
            max_yaw_accel = fast_lim(2);
        else    
            max_yaw_vel = slow_lim(1);
            max_yaw_accel = slow_lim(2);
        end
end

== matlab function Estancia2024_2022a/HORIZON FRAME CONVERSION AND ESTIMATION/Pose Switchbox/Signmoid Type ==
  data: FSM_state input; sigmoid_type output
function sigmoid_type  = sigmoid_type_position(FSM_state)

% QDrone: Position Switchbox
%
% Switching between different sigmoid types based on 
% which state the FSM is in.
%
% v3.0 - 4th October, 2018
%
% INPUTS:
% -------
% FSM_state = current state of the FSM------------------------------------------------------- (#)         [1]
% 
% OUTPUTS:
% --------
% sigmoid_type = an integer whose state determines how the commands/measurements are transformed-- (#)         [1]

% Sigmoid_type = 1; This is for the IDLE, ARM, E_ABORT, E_STOP and DISABLE states of the FSM
% Sigmoid_type = 2; This is for the TAKEOFF THROTTLE state of the FSM
% Sigmoid_type = 3; This is for the FLIGHT state of the FSM
% Sigmoid_type = 4; This is for the TAKEOFF HEIGHT state of the FSM
% Sigmoid_type = 5; This is for the AUTOLAND state of the FSM

sigmoid_type = 0;

switch FSM_state
    case 1 % IDLE STATE
        sigmoid_type = 1;
    case 2 % ARM STATE
        sigmoid_type = 1;
    case 3 % TAKEOFF THROTTLE STATE
        sigmoid_type = 2;
    case 4 % TAKEOFF HEIGHT STATE
        sigmoid_type = 4;
    case 5 % FLIGHT STATE
        sigmoid_type = 3;
    case 6 % AUTOLAND STATE
        sigmoid_type = 5;
    case 7 % EMERGENCY STOP STATE
        sigmoid_type = 1;
    case 8 % EMERGENCY ABORT STATE
        sigmoid_type = 1;
    case 9 % DISABLE STATE
        sigmoid_type = 1;
end

== matlab function Estancia2024_2022a/COMMANDER (ANGLE MODE)/THROTTLE SWITCHBOX /Hover Throttle Sigmoid Parameters ==
  data: sigmoid_type input; enable output; trim_throttle input; takeoff_lim input; land_lim input; throttle_vel input; throttle_ref output; max_throttle_vel output; max_throttle_accel output
function [enable, throttle_ref, max_throttle_vel, max_throttle_accel] = fcn(sigmoid_type, trim_throttle, takeoff_lim, land_lim, throttle_vel)

% Note: Some of the cases below are identical. However, they are separated out 
% based on the states of the state machine for ease of modification in the future. 
% For example, states 4 and 5 are identical. However, if the user wants different 
% signmoid behaviour when taking off than when landing, these cases may not be the same. 

enable = 0;
throttle_ref = 0;
max_throttle_vel = 0;
max_throttle_accel = 0;

switch sigmoid_type
    case 1 % sigmoid = 1 - Command 0 throttle
        % This is for the IDLE, ARM, E_ABORT, and DISABLE states of the FSM
        enable = 0;
        throttle_ref = 0;
        max_throttle_vel = 0;
        max_throttle_accel = 0;

    case 2 % sigmoid = 2 - Sigmoid throttle up from 0 to the trim value
        % This is for the TAKEOFF THROTTLE state of the FSM
        enable = 1;
        throttle_ref = trim_throttle;
        max_throttle_vel = takeoff_lim(1);
        max_throttle_accel = takeoff_lim(2);

    case 3 % sigmoid = 3 - Pass controller throttle straight through + trim value.
        % This is for the TAKEOFF HEIGHT and FLIGHT state of the FSM
        enable = 1;
        throttle_ref = trim_throttle;
        max_throttle_vel = takeoff_lim(1);
        max_throttle_accel = takeoff_lim(2);

    case 4 % sigmoid = 4 - Ignore controller throttle. Sigmoid it down to 0.
        % This is for the E_Landing state of the FSM
        enable = 1;
        throttle_ref = 0;
        if throttle_vel > 0
            max_throttle_vel = takeoff_lim(1);
            max_throttle_accel = takeoff_lim(2);
        else
            max_throttle_vel = land_lim(1);
            max_throttle_accel = land_lim(2);
        end
        
    case 5 % sigmoid = 5 - Pass controller throttle straight through + trim value.
        % This is for the AUTOLAND state of the FSM
        enable = 1;
        throttle_ref = trim_throttle;
        max_throttle_vel = takeoff_lim(1);
        max_throttle_accel = takeoff_lim(2);

end

== matlab function Estancia2024_2022a/COMMANDER (ANGLE MODE)/STATE MACHINE LOGIC ==
  data: E_Abort output; isArm output; pt_ARM_to_TAKEOFF_THROTTLE output; pt_TAKE_OFF_HEIGHT_TO_AUTOLAND output; pt_FLIGHT_TO_AUTOLAND output; current_state input; initializing input; Tracking_Issue input; Communication_Issue input; low_battery input; trigger_1 input; trigger_2 input; E_abort input; joystick_issue input; net_throttle_at_trim input; net_throttle_close_to_zero input; ctrl_throttle_close_to_zero input; take_off_successful input; flying_too_low input; flying_too_high input; close_to_ground input; pt_TAKEOFF_THROTTLE_TO_TAKEOFF_HEIGHT output; pt_TAKE_OFF_HEIGHT_TO_FLIGHT output; pt_AUTOLAND_TO_DISABLE output; pt_EMERGENCY_STOP_TO_DISABLE output; pt_EMERGENCY_ABORT_TO_DISABLE output; Error output; stop_model output; sensor_failed input
function [E_Abort, isArm, pt_ARM_to_TAKEOFF_THROTTLE, pt_TAKE_OFF_HEIGHT_TO_AUTOLAND, pt_FLIGHT_TO_AUTOLAND, pt_TAKEOFF_THROTTLE_TO_TAKEOFF_HEIGHT, pt_TAKE_OFF_HEIGHT_TO_FLIGHT, pt_AUTOLAND_TO_DISABLE, pt_EMERGENCY_STOP_TO_DISABLE, pt_EMERGENCY_ABORT_TO_DISABLE, Error, stop_model]...
    = SM_logic(current_state, initializing, Tracking_Issue, Communication_Issue, low_battery, trigger_1, trigger_2, E_abort, joystick_issue,...
    net_throttle_at_trim, net_throttle_close_to_zero, ctrl_throttle_close_to_zero, take_off_successful, flying_too_low, flying_too_high, close_to_ground, sensor_failed)

% Programmatic Logic Block
%
% Logic for the FSM is generated here based on a variety of signals.
% Mostly, logic to programmatically trigger the transition to either a 
% natural next state, or an Error state, is generated here.
%
% Last modified: March, 2020
%
% INPUTS:
% -------
% current_state = previous state of the FSM-------------------------------------------------- (#)         [1]
% initializing = signal representing that the system is initializing (first 5s + buffer)- - - (bool)      [1]
% comm = communication signal representing MAVLINK connection-------------------------------- (bool)      [1]
% peripheral = signal representing joystick and optitrack connection- - - - - - - - - - - - - (bool)      [2]
% low_battery = signal representing low battery---------------------------------------------- (bool)      [1]
% trigger_1 = trigger representing ARM/DISARM - - - - - - - - - - - - - - - - - - - - - - - - (bool)      [1]
% trigger_2 = trigger representing TAKEOFF/AUTOLAND------------------------------------------ (bool)      [1]
% motors_not_spinning = signal representing the motors not spinning - - - - - - - - - - - - - (bool)      [1]
% net_throttle_at_trim = trim throttle for the application drone ---------------------------- (bool)      [1]
% net_throttle_close_to_zero = net throttle is close to zero in emergency stop mode - - - - - (bool)      [1]
% ctrl_throttle_close_to_zero = ctrl throttle is close to zero in emergency stop mode - - - - (bool)      [1]
% take_off_successful = signal representing whether drone has taken-off successfully -------- (bool)      [1]
% flying_too_low = signal representing whether the drone's height is below threshold and cmd- (bool)      [1]
% flying_too_high = signal representing whether the drone's height is above threshold-------- (bool)      [1]
% close_to_ground = signal representing whether the drone is close to the ground to autoland- (bool)      [1]
% 
% OUTPUTS:
% --------
% Error = Whether an Error is issued or not                                                             (bool)    [1]
% E_Abort = fed through for ease of understanding flow (see STATE MACHINE TRANSITION BLOCK)             (bool)    [1]
% isArm = programmatic transition state                                                                 (bool)    [1]
% takeoff = fed through for ease of understanding flow (see STATE MACHINE TRANSITION BLOCK)             (bool)    [1]
% pt_ARM_to_TAKEOFF_THROTTLE = programmatic transition state BEGIN_STATE_TO_FINAL_STATE                 (bool)    [1]
% pt_TAKEOFF_THROTTLE_TO_TAKEOFF_HEIGHT = programmatic transition state BEGIN_STATE_TO_FINAL_STATE      (bool)    [1]
% pt_TAKE_OFF_HEIGHT_TO_AUTOLAND = programmatic transition state BEGIN_STATE_TO_FINAL_STATE             (bool)    [1]
% pt_TAKEOFF_THROTTLE_TO_TAKEOFF_HEIGHT = programmatic transition state BEGIN_STATE_TO_FINAL_STATE      (bool)    [1]
% pt_TAKE_OFF_HEIGHT_TO_FLIGHT = programmatic transition state BEGIN_STATE_TO_FINAL_STATE               (bool)    [1]
% pt_AUTOLAND_TO_DISABLE = programmatic transition state BEGIN_STATE_TO_FINAL_STATE                     (bool)    [1]
% pt_EMERGENCY_STOP_TO_DISABLE = programmatic transition state BEGIN_STATE_TO_FINAL_STATE               (bool)    [1]
% pt_EMERGENCY_ABORT_TO_DISABLE = programmatic transition state BEGIN_STATE_TO_FINAL_STATE              (bool)    [1]
% stop_model = STOP THE MODEL AFTER                                                                     (bool)    [1]

Error = 0;
E_Abort = E_abort;
isArm = false;
pt_ARM_to_TAKEOFF_THROTTLE = false;
pt_TAKEOFF_THROTTLE_TO_TAKEOFF_HEIGHT = false;
pt_TAKE_OFF_HEIGHT_TO_AUTOLAND = false;
pt_TAKE_OFF_HEIGHT_TO_FLIGHT = false;
pt_FLIGHT_TO_AUTOLAND = false;
pt_AUTOLAND_TO_DISABLE = false;
pt_EMERGENCY_STOP_TO_DISABLE = false;
pt_EMERGENCY_ABORT_TO_DISABLE = false;
stop_model = 0;

switch current_state
    %---------------------------------------------------------------------%
    case 1 % IDLE STATE
        if (Communication_Issue)||...          % Communication issue
           (joystick_issue)||...               % joystick issue
           (Tracking_Issue)||...               % optitrack issue
           (low_battery)||...                  % low batter  
           (sensor_failed)||...                % if sensor (IMU) failure is detected on drone stabilizer    
           ((trigger_1)&&(initializing))||...  % armed while initializing
           (trigger_2)||...                    % tried to takeoff while initializing
           (~ctrl_throttle_close_to_zero)      % if throttle isn't at zero, don't arm
           %----------------------------------------%
            Error = 1;
        elseif trigger_1 % user arms
            isArm = true;
        end
    %---------------------------------------------------------------------%    
    case 2 % ARMED STATE
        isArm = trigger_1;
        if (Communication_Issue)||...          % Communication issue
           (joystick_issue)||...               % joystick issue
           (Tracking_Issue)||...               % optitrack issue
           (low_battery)||...                  % low battery
           (sensor_failed)||...                % if sensor (IMU) failure is detected on drone stabilizer
           (~ctrl_throttle_close_to_zero)      % if throttle isn't at zero, don't arm
           %----------------------------------------%
            Error = 1;
        elseif trigger_1 && trigger_2
            pt_ARM_to_TAKEOFF_THROTTLE = true;
        end        
    %---------------------------------------------------------------------%
    case 3 % TAKEOFF_THROTTLE STATE
        if (Communication_Issue)||...     % Communication issue
           (joystick_issue)||...          % joystick issue
           (Tracking_Issue)||...          % optitrack issue           
           (low_battery)||...             % low battery
           (sensor_failed)||...           % if sensor (IMU) failure is detected on drone stabilizer
           (~trigger_1)||...              % user disarms
           (~trigger_2)||...              % user commands auto-land before drone starts taking off
           (~ctrl_throttle_close_to_zero) % if throttle isn't at zero, don't arm
           %----------------------------------------%
            Error = 1;
        elseif net_throttle_at_trim
            pt_TAKEOFF_THROTTLE_TO_TAKEOFF_HEIGHT = true;
        end
    %---------------------------------------------------------------------%
    case 4 % TAKEOFF_HEIGHT STATE
        if (Communication_Issue)||... % Communication issue
           (joystick_issue)||...      % joystick issue
           (Tracking_Issue)||...      % optitrack issue
           (sensor_failed)||...       % if sensor (IMU) failure is detected on drone stabilizer    
           (flying_too_low)||...      % current height is below safety threshold 
           (flying_too_high)||...     % flying above safety margin (w.r.t optitrack)
           (~trigger_1)               % user disarms
            %----------------------------------------%
            Error = 1;
        elseif (~trigger_2)||low_battery 
            pt_TAKE_OFF_HEIGHT_TO_AUTOLAND = true;
        elseif take_off_successful
            pt_TAKE_OFF_HEIGHT_TO_FLIGHT = true;
        end
    %---------------------------------------------------------------------%
    case 5 % FLIGHT STATE
        if (Communication_Issue)||...   % Communication issue
           (joystick_issue)||...        % joystick issue
           (Tracking_Issue)||...        % optitrack issue
           (sensor_failed)||...         % if sensor (IMU) failure is detected on drone stabilizer
           (flying_too_low)||...        % current height is below safety threshold  
           (flying_too_high)||...       % flying above safety margin (w.r.t optitrack)
           (~trigger_1)                 % user disarms
           %----------------------------------------%
            Error = 1;
        elseif (~trigger_2)||low_battery
            pt_FLIGHT_TO_AUTOLAND = true;
        end
    %---------------------------------------------------------------------%
    case 6 % AUTOLAND STATE
        if (Communication_Issue)||...  % Communication issue
           (joystick_issue)||...       % joystick issue
           (Tracking_Issue)||...       % optitrack issue
           (sensor_failed)||...        % if sensor (IMU) failure is detected on drone stabilizer
           (flying_too_high)||...      % flying above safety margin (w.r.t optitrack)    
           (~trigger_1)                % user disarms
           %----------------------------------------%
            Error = 1;
        elseif close_to_ground 
            pt_AUTOLAND_TO_DISABLE = true;
        end
    %---------------------------------------------------------------------%
    case 7 % EMERGENCY LAND STATE
        if net_throttle_close_to_zero 
            pt_EMERGENCY_STOP_TO_DISABLE = true;
        end
    %---------------------------------------------------------------------%
    case 8 % EMERGENCY ABORT STATE
        pt_EMERGENCY_ABORT_TO_DISABLE = true;
    %---------------------------------------------------------------------%
    case 9
        % Stop the model.
        stop_model = 1;
end

== matlab function Estancia2024_2022a/COMMANDER (ANGLE MODE)/MPC/MPC Z Controller/MATLAB Function ==
  data: u input; y output
function y = fcn(u)

% y = [u(1),u(2),u(3)]';
y = u;
